simulink library "LDM_Controller"  (R2018b)
settings: Solver=VariableStepAuto  StartTime=0.0  StopTime=10.0  RelTol=1e-3
values from neighbouring files (symbols this model uses):
  K10_LDM_aOLCtrlerTableX : value not decoded    [LDM_DataDict.sldd]
  K10_LDM_torqOLCtrlerTableY : value not decoded    [LDM_DataDict.sldd]
  K_LDM_torqDecelClsCtrlerLowLim = -1000.0    [LDM_DataDict.sldd]
  K_LDM_torqDecelClsCtrlerUpLim = 1000.0    [LDM_DataDict.sldd]
  K_LDM_torqDecelCtrlerLowLim = 0.0    [LDM_DataDict.sldd]
  K_LDM_torqDecelCtrlerUpLim = 20000.0    [LDM_DataDict.sldd]
  K_LDM_torqOLCtrlerDecRate = 2.0    [LDM_DataDict.sldd]
  K_LDM_torqOLCtrlerIncRate = 2.0    [LDM_DataDict.sldd]
  K_LDM_torqOLCtrlerLowLim = 0.0    [LDM_DataDict.sldd]
  K_LDM_torqOLCtrlerResetLim = 10.0    [LDM_DataDict.sldd]
  K_LDM_torqOLCtrlerUpLim = 20000.0    [LDM_DataDict.sldd]
  LDM_VLD_EN_T : value not decoded    [LDM_DataDict.sldd]
  LDMCtrlMode_en_t : value not decoded    [LDM_DataDict.sldd]
undefined symbols (not defined in the file or in its folder): DiscIntNeverNeededParam
libraries: simulink x12
(part 1 of 2)
settings Model: Creator=wxmjy  LastModifiedBy=wxmjy

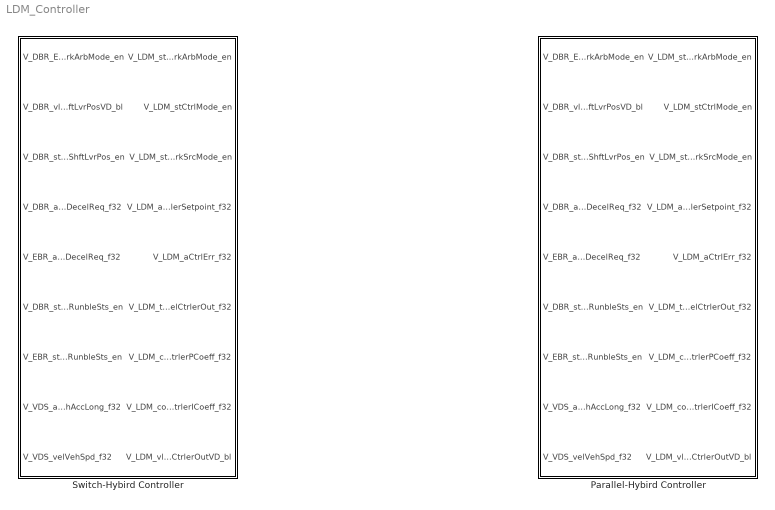
== system LDM_Controller ==
  Parallel-Hybird Controller : Subsystem
  Switch-Hybird Controller : Subsystem

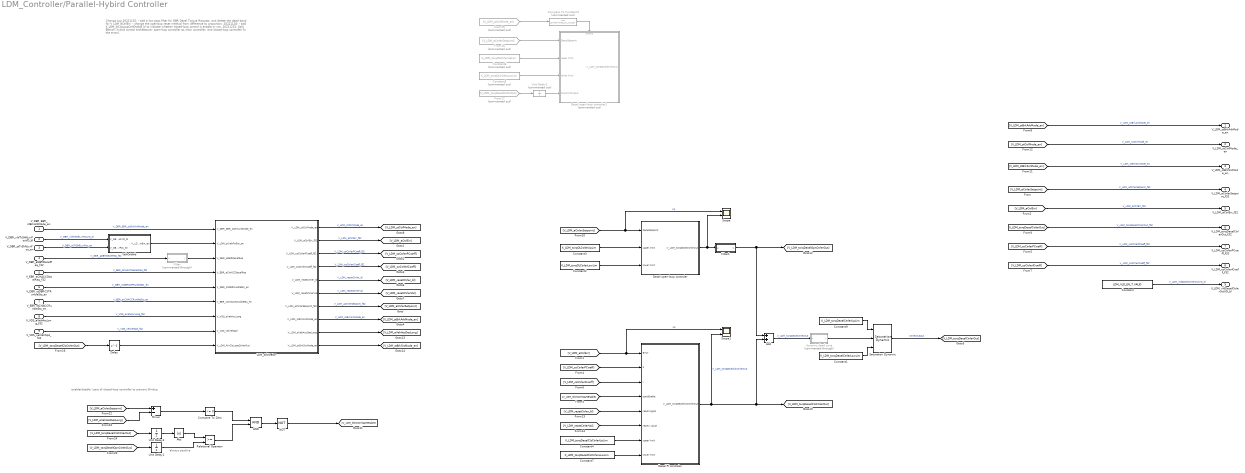
== system LDM_Controller/Parallel-Hybird Controller ==
  note: Change Log
      | 20221125:
      | - add a low-pass filter for DBR Decel Torque Request, and delete the dead band for V_LDM_aCtrlErr;
      | - change the openloop reset method from difference to proportion;
      | 20221128:
      | - add K_LDM_blClsLoopCtrlEnable_bl to indicate whether closed-loop control is enable or not.
      | 20221223:
      | Split Branch: hybrid control architecture: open-loop controller as main controller, and closed-loop controller fix the errors.
  note: always positive
  note: enable/disable I part of closed-loop controller to prevent Windup
  V_DBR_EBR_stBrkArbMode_en : Inport  OutDataTypeStr=Enum: BrkArbMode_en_t
  V_DBR_vldTrShftLvrPosVD_bl : Inport  Port=2
  V_DBR_stTrShftLvrPos_en : Inport  Port=3  OutDataTypeStr=Enum: TrShftLvrPos_en_t
  V_DBR_aDBRDecelReq_f32 : Inport  Port=4
  V_EBR_aCHACCDecelReq_f32 : Inport  Port=5
  V_DBR_stDBRCSTRunbleSts_en : Inport  Port=6  OutDataTypeStr=Enum: DBRCSTRunbleSts_en_t
  V_EBR_stCHACCRunbleSts_en : Inport  Port=7  OutDataTypeStr=Enum: CHACCRunbleSts_en_t
  V_VDS_aVehAccLong_f32 : Inport  Port=8
  V_VDS_velVehSpd_f32 : Inport  Port=9
  AND : Logic  AllPortsSameDT=off  OutDataTypeStr=boolean
  Abs : Abs
  Add : Sum
  Compare To Constant1 : simulink/Logic and Bit Operations/Compare To Constant  Commented=on  relop===  const=LDMCtrlMode_en_t.OLCtrl  OutDataTypeStr=boolean
  Compare To Zero : simulink/Logic and Bit Operations/Compare To Zero  relop=<=  OutDataTypeStr=boolean
  Constant : Constant  Value=LDM_VLD_EN_T.VALID
  Constant1 : Constant  Value=K_LDM_torqDecelCtrlerLowLim  OutDataTypeStr=single
  Constant2 : Constant  Value=K_LDM_torqOLCtrlerLowLim  OutDataTypeStr=single
  Constant3 : Constant  Value=K_LDM_torqOLCtrlerUpLim  OutDataTypeStr=single
  Constant4 : Constant  Value=K_LDM_torqDecelClsCtrlerUpLim  OutDataTypeStr=single
  Constant5 : Constant  Commented=on  Value=K_LDM_torqOLCtrlerLowLim  OutDataTypeStr=single
  Constant6 : Constant  Commented=on  Value=K_LDM_torqOLCtrlerUpLim  OutDataTypeStr=single
  Constant7 : Constant  Value=K_LDM_torqDecelClsCtrlerLowLim  OutDataTypeStr=single
  Constant9 : Constant  Value=K_LDM_torqDecelCtrlerUpLim  OutDataTypeStr=single
  Decel PI controler : Subsystem
  Decel open-loop controler : Subsystem
  Decel open-loop controler1 : Subsystem  Commented=on
  Delay : Delay  DelayLength=1
  Filter : Subsystem  Commented=through
  Filter1 : Subsystem
  From17 : From  Commented=on  GotoTag=V_LDM_torqDecelCtrlerOut
  From18 : From  Commented=on  GotoTag=V_LDM_aCtrlerSetpoint
  From19 : From  Commented=on  GotoTag=V_LDM_stCtrlMode_en
  LDM_Arbitrator : Stateflow chart  TreatAsAtomicUnit=on
  Minus : Sum  Inputs=+-
  NOT : Logic  Operator=NOT  AllPortsSameDT=off  OutDataTypeStr=boolean
  Relational Operator : RelationalOperator  OutDataTypeStr=boolean  RndMeth=Simplest
  Saturation Dynamic : simulink/Discontinuities/Saturation Dynamic  OutMin=[]  OutMax=[]  OutDataTypeStr=single  OutputDataTypeScalingMode=single  OutDataType=fixdt(1, 16)  OutScaling=2^-10  DoSatur=off
  Scope : Scope  NumInputPorts=2
  Scope1 : Scope  NumInputPorts=2
  Unit Delay1 : UnitDelay  SampleTime=-1
  Unit Delay2 : UnitDelay  Commented=on  SampleTime=-1
  Unit Delay3 : UnitDelay  SampleTime=-1
  VehOritArb : Stateflow chart  TreatAsAtomicUnit=on
  dynamic dead zone : Subsystem  Commented=through
  V_LDM_stBrkArbMode_en : Outport
  V_LDM_stCtrlMode_en : Outport  Port=2
  V_LDM_stBrkSrcMode_en : Outport  Port=3
  V_LDM_aCtrlerSetpoint_f32 : Outport  Port=4
  V_LDM_aCtrlErr_f32 : Outport  Port=5
  V_LDM_torqDecelCtrlerOut_f32 : Outport  Port=6
  V_LDM_coCtrlerPCoeff_f32 : Outport  Port=7
  V_LDM_coCtrlerICoeff_f32 : Outport  Port=8
  V_LDM_vldDecelCtrlerOutVD_bl : Outport  Port=9
  wires:
  [V_LDM_stBrkSrcMode_en] -> V_LDM_stBrkSrcMode_en/1  "V_LDM_stBrkSrcMode_en"
  LDM_Arbitrator/10(V_LDM_stBrkSrcMode_en) -> [V_LDM_stBrkSrcMode_en]
  LDM_Arbitrator/9(V_LDM_aVehAccDecLong) -> [V_LDM_aVehAccDecLong]
  Relational Operator/1 -> AND/2
  Compare To Zero/1 -> AND/1
  Minus/1 -> Compare To Zero/1
  [V_LDM_aVehAccDecLong] -> Minus/2
  [V_LDM_aCtrlerSetpoint] -> Minus/1
  NOT/1 -> [V_LDM_blClsCtrlIpartEnable]
  Abs/1 -> Relational Operator/1
  Unit Delay1/1 -> Relational Operator/2
  Unit Delay3/1 -> Abs/1
  [V_LDM_torqDecelClsCtrlerOut] -> Unit Delay3/1
  [V_LDM_torqDecelOpnCtrlerOut] -> Unit Delay1/1
  [V_LDM_blClsCtrlIpartEnable] -> Decel PI controler/4(IpartEnable)
  AND/1 -> NOT/1
  Filter1/1(y) -> Add/1, [V_LDM_torqDecelOpnCtrlerOut]
  Constant/1 -> V_LDM_vldDecelCtrlerOutVD_bl/1  "V_LDM_vldDecelCtrlerOutVD_bl"
  [V_LDM_coCtrlerPCoeff] -> Decel PI controler/2(P)
  Saturation Dynamic/1 -> [V_LDM_torqDecelCtrlerOut]  "CtrlerOutput"
  Constant1/1 -> Saturation Dynamic/3
  Constant9/1 -> Saturation Dynamic/1
  Decel open-loop controler/1(V_LDM_torqDecelCtrlerOut) -> Filter1/1(u), Scope/2
  Decel PI controler/1(V_LDM_torqDecelClsCtrlerOut) -> [V_LDM_torqDecelClsCtrlerOut], Add/2, Scope1/2  "V_LDM_torqDecelClsCtrlerOut"
  [V_LDM_aCtrlErr] -> Decel PI controler/1(Error), Scope1/1  "sp"
  [V_LDM_stBrkArbMode_en] -> V_LDM_stBrkArbMode_en/1  "V_LDM_stBrkArbMode_en"
  LDM_Arbitrator/6(V_LDM_resetCtrlerVal) -> [V_LDM_resetCtrlerVal]  "V_LDM_resetCtrlerVal"
  [V_LDM_coCtrlerICoeff] -> V_LDM_coCtrlerICoeff_f32/1  "V_LDM_coCtrlerICoeff_f32"
  Filter/1(y) -> LDM_Arbitrator/3(V_DBR_aDBRDecelReq)
  [V_LDM_stCtrlMode_en] -> V_LDM_stCtrlMode_en/1  "V_LDM_stCtrlMode_en"
  dynamic dead zone/1(y) -> Saturation Dynamic/2
  [V_LDM_aCtrlerSetpoint] -> Decel open-loop controler/1(DecelSetpoint), Scope/1  "sp"
  [V_LDM_aCtrlerSetpoint] -> V_LDM_aCtrlerSetpoint_f32/1  "V_LDM_aCtrlerSetpoint_f32"
  Constant7/1 -> Decel PI controler/8(lower limit)
  V_DBR_stDBRCSTRunbleSts_en/1 -> LDM_Arbitrator/5(V_DBR_stDBRRunbleSts_en)  "V_DBR_stDBRCSTRunbleSts_en"
  LDM_Arbitrator/2(V_LDM_aCtrlErr_f32) -> [V_LDM_aCtrlErr]  "V_LDM_aCtrlErr_f32"
  LDM_Arbitrator/8(V_LDM_stBrkArbMode_en) -> [V_LDM_stBrkArbMode_en]  "V_LDM_stBrkArbMode_en"
  V_VDS_aVehAccLong_f32/1 -> LDM_Arbitrator/7(V_VDS_aVehAccLong)  "V_VDS_aVehAccLong_f32"
  V_DBR_EBR_stBrkArbMode_en/1 -> LDM_Arbitrator/1(V_DBR_EBR_stBrkArbMode_en)  "V_DBR_EBR_stBrkArbMode_en"
  [V_LDM_torqDecelClsCtrlerOut] -> Delay/1
  [V_LDM_resetCtrlerVal] -> Decel PI controler/6(reset I value)
  V_VDS_velVehSpd_f32/1 -> LDM_Arbitrator/8(V_VDS_velVehSpd)  "V_VDS_velVehSpd_f32"
  Add/1 -> dynamic dead zone/1(u)  "V_LDM_torqDecelCtrlerOut"
  LDM_Arbitrator/1(V_LDM_stCtrlMode_en) -> [V_LDM_stCtrlMode_en]  "V_LDM_stCtrlMode_en"
  V_DBR_stTrShftLvrPos_en/1 -> VehOritArb/2(V_DBR_stTrShftLvrPos_en)  "V_DBR_stTrShftLvrPos_en"
  V_EBR_stCHACCRunbleSts_en/1 -> LDM_Arbitrator/6(V_EBR_stCHACCRunbleSts_en)  "V_EBR_stCHACCRunbleSts_en"
  VehOritArb/1(V_LDM_stVehFwBw_en) -> LDM_Arbitrator/2(V_LDM_stVehFwBw_en)
  Constant4/1 -> Decel PI controler/7(upper limit)
  V_DBR_vldTrShftLvrPosVD_bl/1 -> VehOritArb/1(V_DBR_vldTrShftLvrPosVD_bl)  "V_DBR_vldTrShftLvrPosVD_bl"
  Delay/1 -> LDM_Arbitrator/9(V_LDM_PrvClsLoopCtrlerOut)
  V_DBR_aDBRDecelReq_f32/1 -> Filter/1(u)  "V_DBR_aDBRDecelReq_f32"
  [V_LDM_resetCtrler_bl] -> Decel PI controler/5(reset signal)
  LDM_Arbitrator/3(V_LDM_coCtrlerPCoeff_f32) -> [V_LDM_coCtrlerPCoeff]  "V_LDM_coCtrlerPCoeff_f32"
  Constant2/1 -> Decel open-loop controler/3(lower limit)
  LDM_Arbitrator/4(V_LDM_coCtrlerICoeff_f32) -> [V_LDM_coCtrlerICoeff]  "V_LDM_coCtrlerICoeff_f32"
  [V_LDM_coCtrlerPCoeff] -> V_LDM_coCtrlerPCoeff_f32/1  "V_LDM_coCtrlerPCoeff_f32"
  [V_LDM_aCtrlErr] -> V_LDM_aCtrlErr_f32/1  "V_LDM_aCtrlErr_f32"
  Constant3/1 -> Decel open-loop controler/2(upper limit)
  LDM_Arbitrator/5(V_LDM_resetCtrler_bl) -> [V_LDM_resetCtrler_bl]  "V_LDM_resetCtrler_bl"
  [V_LDM_torqDecelCtrlerOut] -> V_LDM_torqDecelCtrlerOut_f32/1  "V_LDM_torqDecelCtrlerOut_f32"
  V_EBR_aCHACCDecelReq_f32/1 -> LDM_Arbitrator/4(V_EBR_aCHACCDecelReq)  "V_EBR_aCHACCDecelReq_f32"
  LDM_Arbitrator/7(V_LDM_aCtrlerSetpoint_f32) -> [V_LDM_aCtrlerSetpoint]  "V_LDM_aCtrlerSetpoint_f32"
  [V_LDM_coCtrlerICoeff] -> Decel PI controler/3(I)
  Constant6/1 -> Decel open-loop controler1/2(upper limit)
  Constant5/1 -> Decel open-loop controler1/3(lower limit)
  Unit Delay2/1 -> Decel open-loop controler1/4(PrevCtrlOutput)
  From19/1 -> Compare To Constant1/1
  From17/1 -> Unit Delay2/1
  Compare To Constant1/1 -> Decel open-loop controler1/Enable
  From18/1 -> Decel open-loop controler1/1(DecelSetpoint)

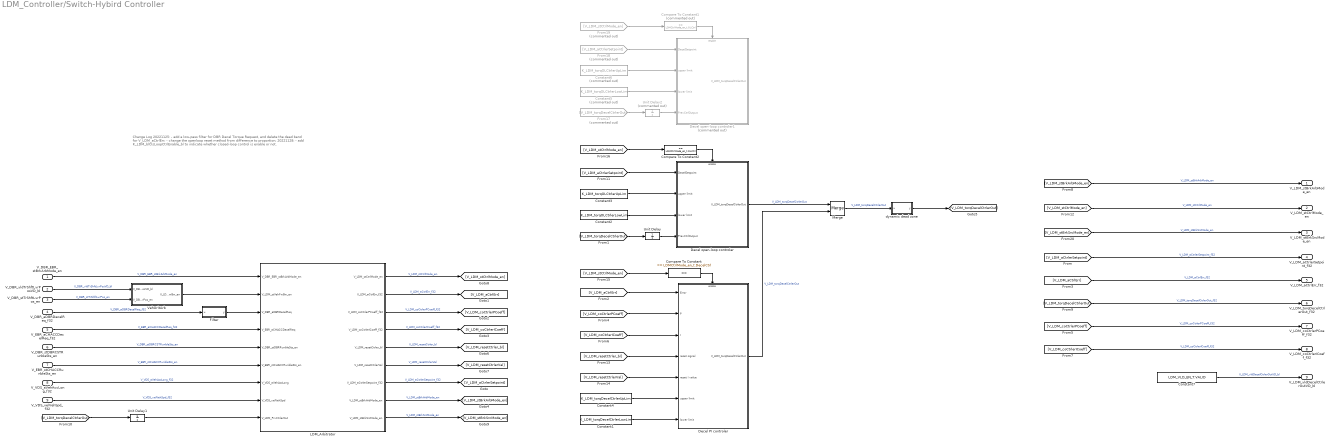
== system LDM_Controller/Switch-Hybird Controller ==
  note: Change Log
      | 20221125:
      | - add a low-pass filter for DBR Decel Torque Request, and delete the dead band for V_LDM_aCtrlErr;
      | - change the openloop reset method from difference to proportion;
      | 20221128:
      | - add K_LDM_blClsLoopCtrlEnable_bl to indicate whether closed-loop control is enable or not.
  V_DBR_EBR_stBrkArbMode_en : Inport  OutDataTypeStr=Enum: BrkArbMode_en_t
  V_DBR_vldTrShftLvrPosVD_bl : Inport  Port=2
  V_DBR_stTrShftLvrPos_en : Inport  Port=3  OutDataTypeStr=Enum: TrShftLvrPos_en_t
  V_DBR_aDBRDecelReq_f32 : Inport  Port=4
  V_EBR_aCHACCDecelReq_f32 : Inport  Port=5
  V_DBR_stDBRCSTRunbleSts_en : Inport  Port=6  OutDataTypeStr=Enum: DBRCSTRunbleSts_en_t
  V_EBR_stCHACCRunbleSts_en : Inport  Port=7  OutDataTypeStr=Enum: CHACCRunbleSts_en_t
  V_VDS_aVehAccLong_f32 : Inport  Port=8
  V_VDS_velVehSpd_f32 : Inport  Port=9
  Compare To Constant : simulink/Logic and Bit Operations/Compare To Constant  relop===  const=LDMCtrlMode_en_t.DecelCtrl  OutDataTypeStr=boolean
  Compare To Constant1 : simulink/Logic and Bit Operations/Compare To Constant  Commented=on  relop===  const=LDMCtrlMode_en_t.OLCtrl  OutDataTypeStr=boolean
  Compare To Constant2 : simulink/Logic and Bit Operations/Compare To Constant  relop===  const=LDMCtrlMode_en_t.OLCtrl  OutDataTypeStr=boolean
  Constant1 : Constant  Value=K_LDM_torqDecelCtrlerLowLim  OutDataTypeStr=single
  Constant2 : Constant  Value=K_LDM_torqOLCtrlerLowLim  OutDataTypeStr=single
  Constant3 : Constant  Value=K_LDM_torqOLCtrlerUpLim  OutDataTypeStr=single
  Constant4 : Constant  Value=K_LDM_torqDecelCtrlerUpLim  OutDataTypeStr=single
  Constant5 : Constant  Commented=on  Value=K_LDM_torqOLCtrlerLowLim  OutDataTypeStr=single
  Constant6 : Constant  Commented=on  Value=K_LDM_torqOLCtrlerUpLim  OutDataTypeStr=single
  Constant7 : Constant  Value=LDM_VLD_EN_T.VALID
  Decel PI controler : Subsystem
  Decel open-loop controler : Subsystem
  Decel open-loop controler1 : Subsystem  Commented=on
  Filter : Subsystem
  From17 : From  Commented=on  GotoTag=V_LDM_torqDecelCtrlerOut
  From18 : From  Commented=on  GotoTag=V_LDM_aCtrlerSetpoint
  From19 : From  Commented=on  GotoTag=V_LDM_stCtrlMode_en
  LDM_Arbitrator : Stateflow chart  TreatAsAtomicUnit=on
  Merge : Merge
  Unit Delay : UnitDelay  SampleTime=-1
  Unit Delay1 : UnitDelay  SampleTime=-1
  Unit Delay2 : UnitDelay  Commented=on  SampleTime=-1
  VehOritArb : Stateflow chart  TreatAsAtomicUnit=on
  dynamic dead zone : Subsystem
  V_LDM_stBrkArbMode_en : Outport
  V_LDM_stCtrlMode_en : Outport  Port=2
  V_LDM_stBrkSrcMode_en : Outport  Port=3
  V_LDM_aCtrlerSetpoint_f32 : Outport  Port=4
  V_LDM_aCtrlErr_f32 : Outport  Port=5
  V_LDM_torqDecelCtrlerOut_f32 : Outport  Port=6
  V_LDM_coCtrlerPCoeff_f32 : Outport  Port=7
  V_LDM_coCtrlerICoeff_f32 : Outport  Port=8
  V_LDM_vldDecelCtrlerOutVD_bl : Outport  Port=9
  wires:
  LDM_Arbitrator/9(V_LDM_stBrkSrcMode_en) -> [V_LDM_stBrkSrcMode_en]  "V_LDM_stBrkSrcMode_en"
  [V_LDM_stBrkSrcMode_en] -> V_LDM_stBrkSrcMode_en/1  "V_LDM_stBrkSrcMode_en"
  Constant7/1 -> V_LDM_vldDecelCtrlerOutVD_bl/1  "V_LDM_vldDecelCtrlerOutVD_bl"
  From18/1 -> Decel open-loop controler1/1(DecelSetpoint)
  Compare To Constant1/1 -> Decel open-loop controler1/Enable
  From17/1 -> Unit Delay2/1
  From19/1 -> Compare To Constant1/1
  Unit Delay2/1 -> Decel open-loop controler1/4(PrevCtrlOutput)
  Constant5/1 -> Decel open-loop controler1/3(lower limit)
  Constant6/1 -> Decel open-loop controler1/2(upper limit)
  [V_LDM_coCtrlerICoeff] -> Decel PI controler/3(I)
  LDM_Arbitrator/7(V_LDM_aCtrlerSetpoint_f32) -> [V_LDM_aCtrlerSetpoint]  "V_LDM_aCtrlerSetpoint_f32"
  V_EBR_aCHACCDecelReq_f32/1 -> LDM_Arbitrator/4(V_EBR_aCHACCDecelReq)  "V_EBR_aCHACCDecelReq_f32"
  [V_LDM_torqDecelCtrlerOut] -> V_LDM_torqDecelCtrlerOut_f32/1  "V_LDM_torqDecelCtrlerOut_f32"
  LDM_Arbitrator/5(V_LDM_resetCtrler_bl) -> [V_LDM_resetCtrler_bl]  "V_LDM_resetCtrler_bl"
  [V_LDM_stCtrlMode_en] -> Compare To Constant/1
  Constant3/1 -> Decel open-loop controler/2(upper limit)
  [V_LDM_aCtrlErr] -> Decel PI controler/1(Error)
  [V_LDM_aCtrlErr] -> V_LDM_aCtrlErr_f32/1  "V_LDM_aCtrlErr_f32"
  [V_LDM_coCtrlerPCoeff] -> V_LDM_coCtrlerPCoeff_f32/1  "V_LDM_coCtrlerPCoeff_f32"
  [V_LDM_coCtrlerICoeff] -> V_LDM_coCtrlerICoeff_f32/1  "V_LDM_coCtrlerICoeff_f32"
  LDM_Arbitrator/4(V_LDM_coCtrlerICoeff_f32) -> [V_LDM_coCtrlerICoeff]  "V_LDM_coCtrlerICoeff_f32"
  [V_LDM_coCtrlerPCoeff] -> Decel PI controler/2(P)
  Constant2/1 -> Decel open-loop controler/3(lower limit)
  LDM_Arbitrator/3(V_LDM_coCtrlerPCoeff_f32) -> [V_LDM_coCtrlerPCoeff]  "V_LDM_coCtrlerPCoeff_f32"
  [V_LDM_resetCtrler_bl] -> Decel PI controler/4(reset signal)
  V_DBR_aDBRDecelReq_f32/1 -> Filter/1(u)  "V_DBR_aDBRDecelReq_f32"
  Merge/1 -> dynamic dead zone/1(u)  "V_LDM_torqDecelCtrlerOut"
  Unit Delay1/1 -> LDM_Arbitrator/9(V_LDM_PrvCtrlerOut)
  V_DBR_vldTrShftLvrPosVD_bl/1 -> VehOritArb/1(V_DBR_vldTrShftLvrPosVD_bl)  "V_DBR_vldTrShftLvrPosVD_bl"
  Constant4/1 -> Decel PI controler/6(upper limit)
  VehOritArb/1(V_LDM_stVehFwBw_en) -> LDM_Arbitrator/2(V_LDM_stVehFwBw_en)
  V_EBR_stCHACCRunbleSts_en/1 -> LDM_Arbitrator/6(V_EBR_stCHACCRunbleSts_en)  "V_EBR_stCHACCRunbleSts_en"
  V_DBR_stTrShftLvrPos_en/1 -> VehOritArb/2(V_DBR_stTrShftLvrPos_en)  "V_DBR_stTrShftLvrPos_en"
  LDM_Arbitrator/1(V_LDM_stCtrlMode_en) -> [V_LDM_stCtrlMode_en]  "V_LDM_stCtrlMode_en"
  Unit Delay/1 -> Decel open-loop controler/4(PrevCtrlOutput)
  Decel PI controler/1(V_LDM_torqDecelCtrlerOut) -> Merge/2  "V_LDM_torqDecelCtrlerOut"
  V_VDS_velVehSpd_f32/1 -> LDM_Arbitrator/8(V_VDS_velVehSpd)  "V_VDS_velVehSpd_f32"
  [V_LDM_resetCtrlerVal] -> Decel PI controler/5(reset I value)
  [V_LDM_torqDecelCtrlerOut] -> Unit Delay1/1
  Decel open-loop controler/1(V_LDM_torqDecelCtrlerOut) -> Merge/1  "V_LDM_torqDecelCtrlerOut"
  V_DBR_EBR_stBrkArbMode_en/1 -> LDM_Arbitrator/1(V_DBR_EBR_stBrkArbMode_en)  "V_DBR_EBR_stBrkArbMode_en"
  [V_LDM_stCtrlMode_en] -> Compare To Constant2/1
  [V_LDM_torqDecelCtrlerOut] -> Unit Delay/1
  V_VDS_aVehAccLong_f32/1 -> LDM_Arbitrator/7(V_VDS_aVehAccLong)  "V_VDS_aVehAccLong_f32"
  LDM_Arbitrator/8(V_LDM_stBrkArbMode_en) -> [V_LDM_stBrkArbMode_en]  "V_LDM_stBrkArbMode_en"
  LDM_Arbitrator/2(V_LDM_aCtrlErr_f32) -> [V_LDM_aCtrlErr]  "V_LDM_aCtrlErr_f32"
  V_DBR_stDBRCSTRunbleSts_en/1 -> LDM_Arbitrator/5(V_DBR_stDBRRunbleSts_en)  "V_DBR_stDBRCSTRunbleSts_en"
  Compare To Constant/1 -> Decel PI controler/Enable
  Constant1/1 -> Decel PI controler/7(lower limit)
  Compare To Constant2/1 -> Decel open-loop controler/Enable
  [V_LDM_aCtrlerSetpoint] -> V_LDM_aCtrlerSetpoint_f32/1  "V_LDM_aCtrlerSetpoint_f32"
  [V_LDM_aCtrlerSetpoint] -> Decel open-loop controler/1(DecelSetpoint)
  dynamic dead zone/1(y) -> [V_LDM_torqDecelCtrlerOut]
  [V_LDM_stCtrlMode_en] -> V_LDM_stCtrlMode_en/1  "V_LDM_stCtrlMode_en"
  Filter/1(y) -> LDM_Arbitrator/3(V_DBR_aDBRDecelReq)
  LDM_Arbitrator/6(V_LDM_resetCtrlerVal) -> [V_LDM_resetCtrlerVal]  "V_LDM_resetCtrlerVal"
  [V_LDM_stBrkArbMode_en] -> V_LDM_stBrkArbMode_en/1  "V_LDM_stBrkArbMode_en"

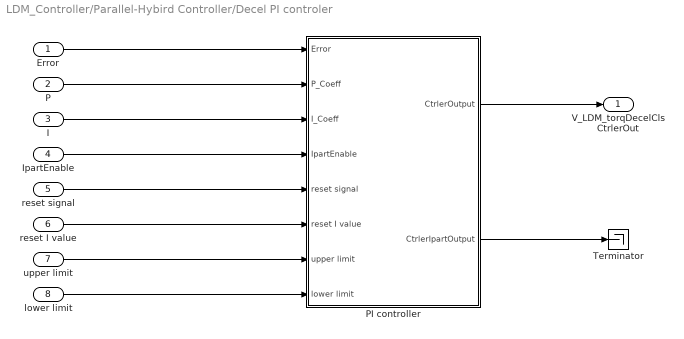
== system LDM_Controller/Parallel-Hybird Controller/Decel PI controler ==
  Error : Inport
  P : Inport  Port=2
  I : Inport  Port=3
  IpartEnable : Inport  Port=4
  reset signal : Inport  Port=5
  reset I value : Inport  Port=6
  upper limit : Inport  Port=7
  lower limit : Inport  Port=8
  PI controller : Subsystem
  Terminator : Terminator
  V_LDM_torqDecelClsCtrlerOut : Outport
  wires:
  IpartEnable/1 -> PI controller/4(IpartEnable)
  PI controller/2(CtrlerIpartOutput) -> Terminator/1
  Error/1 -> PI controller/1(Error)
  P/1 -> PI controller/2(P_Coeff)
  I/1 -> PI controller/3(I_Coeff)
  reset signal/1 -> PI controller/5(reset signal)
  reset I value/1 -> PI controller/6(reset I value)
  PI controller/1(CtrlerOutput) -> V_LDM_torqDecelClsCtrlerOut/1
  lower limit/1 -> PI controller/8(lower limit)
  upper limit/1 -> PI controller/7(upper limit)

== system LDM_Controller/Parallel-Hybird Controller/Decel open-loop controler ==
  DecelSetpoint : Inport
  upper limit : Inport  Port=2
  lower limit : Inport  Port=3
  2-D Lookup Table1 : Lookup_n-D  NumberOfTableDimensions=1  BreakpointsForDimension1=K10_LDM_aOLCtrlerTableX  BreakpointsForDimension2=[0.1,0.2,0.3]  Table=K10_LDM_torqOLCtrlerTableY  InternalRulePriority=Speed  RndMeth=Simplest  InputSameDT=on
  Saturation Dynamic : simulink/Discontinuities/Saturation Dynamic  OutMin=[]  OutMax=[]  OutDataTypeStr=single  OutputDataTypeScalingMode=single  OutDataType=fixdt(1, 16)  OutScaling=2^-10  DoSatur=off
  Signal Conversion : SignalConversion  OverrideOpt=off
  V_LDM_torqDecelCtrlerOut : Outport
  wires:
  DecelSetpoint/1 -> 2-D Lookup Table1/1
  upper limit/1 -> Saturation Dynamic/1
  lower limit/1 -> Saturation Dynamic/3
  Saturation Dynamic/1 -> Signal Conversion/1
  Signal Conversion/1 -> V_LDM_torqDecelCtrlerOut/1
  2-D Lookup Table1/1 -> Saturation Dynamic/2

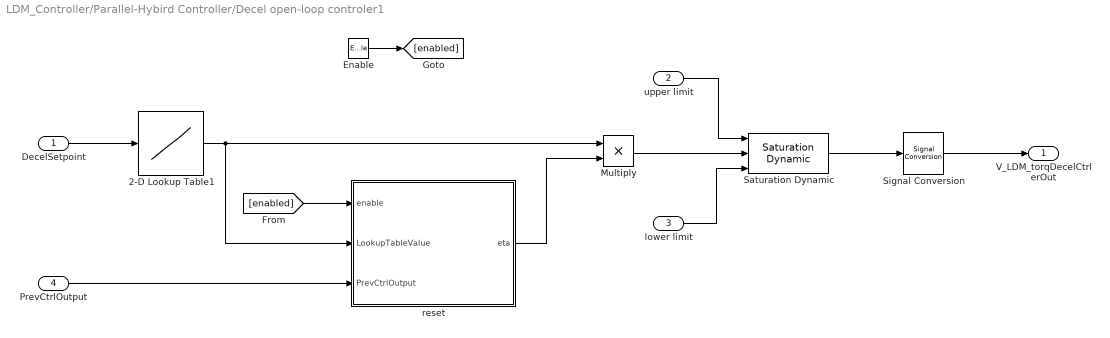
== system LDM_Controller/Parallel-Hybird Controller/Decel open-loop controler1 ==
  DecelSetpoint : Inport
  upper limit : Inport  Port=2
  lower limit : Inport  Port=3
  PrevCtrlOutput : Inport  Port=4
  Enable : EnablePort  ShowOutputPort=on
  2-D Lookup Table1 : Lookup_n-D  NumberOfTableDimensions=1  BreakpointsForDimension1=K10_LDM_aOLCtrlerTableX  BreakpointsForDimension2=[0.1,0.2,0.3]  Table=K10_LDM_torqOLCtrlerTableY  InternalRulePriority=Speed  RndMeth=Simplest  InputSameDT=on
  Multiply : Product
  Saturation Dynamic : simulink/Discontinuities/Saturation Dynamic  OutMin=[]  OutMax=[]  OutDataTypeStr=single  OutputDataTypeScalingMode=single  OutDataType=fixdt(1, 16)  OutScaling=2^-10  DoSatur=off
  Signal Conversion : SignalConversion  OverrideOpt=off
  reset : Stateflow chart  TreatAsAtomicUnit=on
  V_LDM_torqDecelCtrlerOut : Outport
  wires:
  [enabled] -> reset/1(enable)
  Multiply/1 -> Saturation Dynamic/2
  reset/1(eta) -> Multiply/2
  PrevCtrlOutput/1 -> reset/3(PrevCtrlOutput)
  Enable/1 -> [enabled]
  DecelSetpoint/1 -> 2-D Lookup Table1/1
  Signal Conversion/1 -> V_LDM_torqDecelCtrlerOut/1
  Saturation Dynamic/1 -> Signal Conversion/1
  lower limit/1 -> Saturation Dynamic/3
  upper limit/1 -> Saturation Dynamic/1
  2-D Lookup Table1/1 -> reset/2(LookupTableValue), Multiply/1

== system LDM_Controller/Parallel-Hybird Controller/Filter ==
  u : Inport
  Add : Sum
  Constant1 : Constant  Value=0.5  OutDataTypeStr=single
  Constant2 : Constant  OutDataTypeStr=single
  Minus : Sum  Inputs=+-
  Multiply : Product
  Multiply1 : Product
  Unit Delay : UnitDelay  SampleTime=-1
  y : Outport
  wires:
  Constant2/1 -> Minus/1
  Minus/1 -> Multiply1/2
  Add/1 -> y/1, Unit Delay/1  "y"
  Unit Delay/1 -> Multiply/2  "y_k-1"
  Multiply1/1 -> Add/1
  Multiply/1 -> Add/2
  Constant1/1 -> Multiply/1, Minus/2
  u/1 -> Multiply1/1

== system LDM_Controller/Parallel-Hybird Controller/Filter1 ==
  u : Inport
  Add : Sum
  Constant1 : Constant  Value=0.7  OutDataTypeStr=single
  Constant2 : Constant  Value=0.3  OutDataTypeStr=single
  Multiply : Product
  Multiply1 : Product
  Unit Delay : UnitDelay  SampleTime=-1
  y : Outport
  wires:
  Constant2/1 -> Multiply1/2
  Add/1 -> y/1, Unit Delay/1  "y"
  Unit Delay/1 -> Multiply/2  "y_k-1"
  Multiply1/1 -> Add/1
  Multiply/1 -> Add/2
  Constant1/1 -> Multiply/1
  u/1 -> Multiply1/1

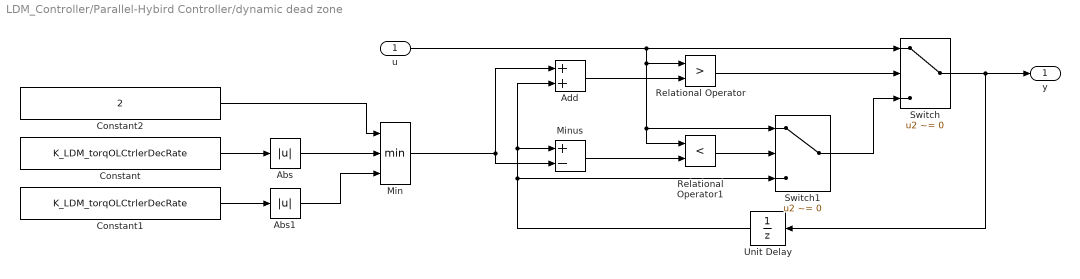
== system LDM_Controller/Parallel-Hybird Controller/dynamic dead zone ==
  u : Inport
  Abs : Abs
  Abs1 : Abs
  Add : Sum
  Constant : Constant  Value=K_LDM_torqOLCtrlerDecRate  OutDataTypeStr=single
  Constant1 : Constant  Value=K_LDM_torqOLCtrlerDecRate  OutDataTypeStr=single
  Constant2 : Constant  Value=2  OutDataTypeStr=single
  Min : MinMax  Inputs=3
  Minus : Sum  Inputs=+-
  Relational Operator : RelationalOperator  Operator=>  OutDataTypeStr=boolean  RndMeth=Simplest
  Relational Operator1 : RelationalOperator  Operator=<  OutDataTypeStr=boolean  RndMeth=Simplest
  Switch : Switch  Criteria=u2 ~= 0
  Switch1 : Switch  Criteria=u2 ~= 0
  Unit Delay : UnitDelay  SampleTime=-1
  y : Outport
  wires:
  Switch/1 -> Unit Delay/1, y/1
  u/1 -> Switch/1, Relational Operator1/1, Switch1/1, Relational Operator/1
  Unit Delay/1 -> Minus/1, Add/2, Switch1/3
  Constant/1 -> Abs/1
  Add/1 -> Relational Operator/2
  Minus/1 -> Relational Operator1/2
  Relational Operator/1 -> Switch/2
  Relational Operator1/1 -> Switch1/2
  Switch1/1 -> Switch/3
  Min/1 -> Add/1, Minus/2
  Constant1/1 -> Abs1/1
  Abs/1 -> Min/2
  Abs1/1 -> Min/3
  Constant2/1 -> Min/1

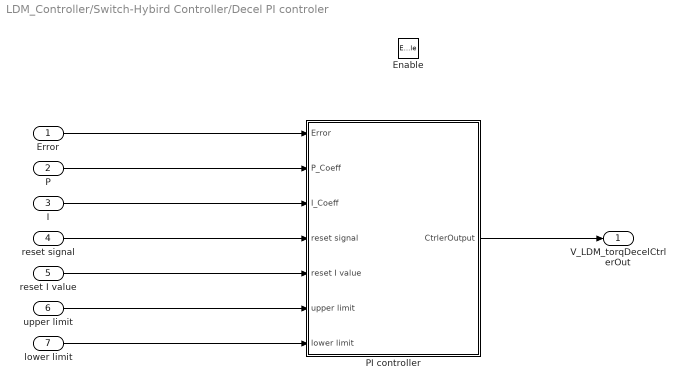
== system LDM_Controller/Switch-Hybird Controller/Decel PI controler ==
  Error : Inport
  P : Inport  Port=2
  I : Inport  Port=3
  reset signal : Inport  Port=4
  reset I value : Inport  Port=5
  upper limit : Inport  Port=6
  lower limit : Inport  Port=7
  Enable : EnablePort
  PI controller : Subsystem
  V_LDM_torqDecelCtrlerOut : Outport
  wires:
  upper limit/1 -> PI controller/6(upper limit)
  lower limit/1 -> PI controller/7(lower limit)
  PI controller/1(CtrlerOutput) -> V_LDM_torqDecelCtrlerOut/1
  reset I value/1 -> PI controller/5(reset I value)
  reset signal/1 -> PI controller/4(reset signal)
  I/1 -> PI controller/3(I_Coeff)
  P/1 -> PI controller/2(P_Coeff)
  Error/1 -> PI controller/1(Error)

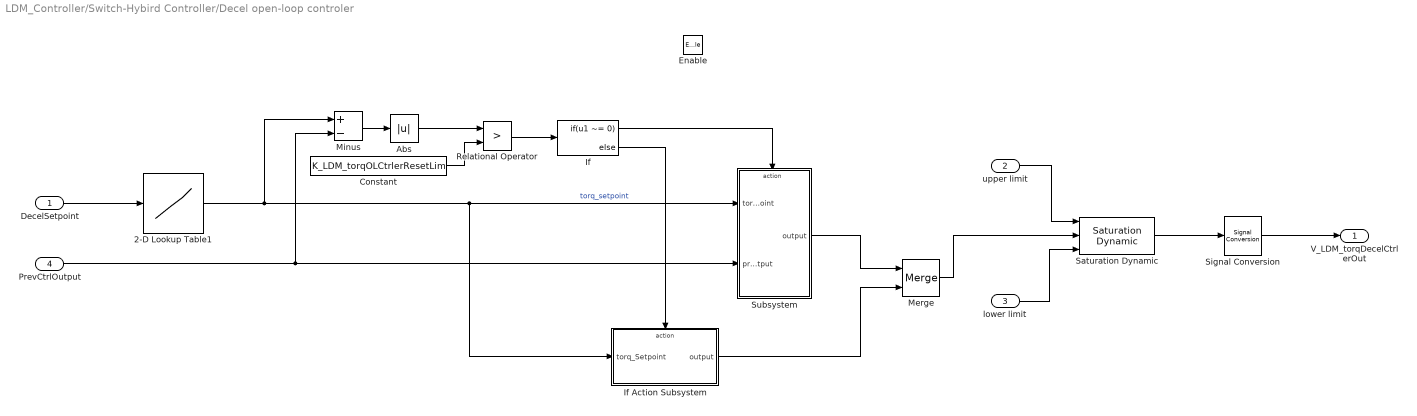
== system LDM_Controller/Switch-Hybird Controller/Decel open-loop controler ==
  DecelSetpoint : Inport
  upper limit : Inport  Port=2
  lower limit : Inport  Port=3
  PrevCtrlOutput : Inport  Port=4
  Enable : EnablePort
  2-D Lookup Table1 : Lookup_n-D  NumberOfTableDimensions=1  BreakpointsForDimension1=K10_LDM_aOLCtrlerTableX  BreakpointsForDimension2=[0.1,0.2,0.3]  Table=K10_LDM_torqOLCtrlerTableY  InternalRulePriority=Speed  RndMeth=Simplest  InputSameDT=on
  Abs : Abs
  Constant : Constant  Value=K_LDM_torqOLCtrlerResetLim  OutDataTypeStr=single
  If : If  IfExpression=u1 ~= 0
  If Action Subsystem : Subsystem  TreatAsAtomicUnit=on
  Merge : Merge
  Minus : Sum  Inputs=+-
  Relational Operator : RelationalOperator  Operator=>  OutDataTypeStr=boolean  RndMeth=Simplest
  Saturation Dynamic : simulink/Discontinuities/Saturation Dynamic  OutMin=[]  OutMax=[]  OutDataTypeStr=single  OutputDataTypeScalingMode=single  OutDataType=fixdt(1, 16)  OutScaling=2^-10  DoSatur=off
  Signal Conversion : SignalConversion  OverrideOpt=off
  Subsystem : Subsystem
  V_LDM_torqDecelCtrlerOut : Outport
  wires:
  If Action Subsystem/1(output) -> Merge/2
  Subsystem/1(output) -> Merge/1
  If/2 -> If Action Subsystem/Action
  Constant/1 -> Relational Operator/2
  Relational Operator/1 -> If/1
  If/1 -> Subsystem/Action
  Merge/1 -> Saturation Dynamic/2
  Abs/1 -> Relational Operator/1
  Minus/1 -> Abs/1
  2-D Lookup Table1/1 -> Subsystem/1(torq_setpoint), If Action Subsystem/1(torq_Setpoint), Minus/1  "torq_setpoint"
  PrevCtrlOutput/1 -> Subsystem/2(prevOutput), Minus/2
  Signal Conversion/1 -> V_LDM_torqDecelCtrlerOut/1
  Saturation Dynamic/1 -> Signal Conversion/1
  lower limit/1 -> Saturation Dynamic/3
  upper limit/1 -> Saturation Dynamic/1
  DecelSetpoint/1 -> 2-D Lookup Table1/1

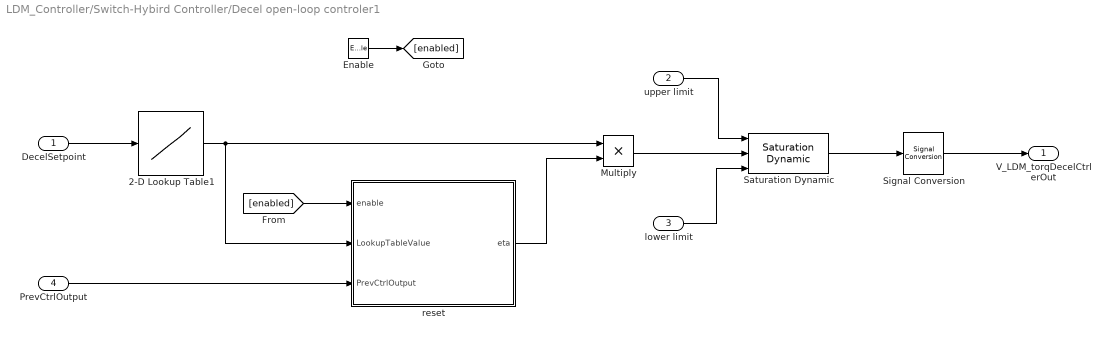
== system LDM_Controller/Switch-Hybird Controller/Decel open-loop controler1 ==
  DecelSetpoint : Inport
  upper limit : Inport  Port=2
  lower limit : Inport  Port=3
  PrevCtrlOutput : Inport  Port=4
  Enable : EnablePort  ShowOutputPort=on
  2-D Lookup Table1 : Lookup_n-D  NumberOfTableDimensions=1  BreakpointsForDimension1=K10_LDM_aOLCtrlerTableX  BreakpointsForDimension2=[0.1,0.2,0.3]  Table=K10_LDM_torqOLCtrlerTableY  InternalRulePriority=Speed  RndMeth=Simplest  InputSameDT=on
  Multiply : Product
  Saturation Dynamic : simulink/Discontinuities/Saturation Dynamic  OutMin=[]  OutMax=[]  OutDataTypeStr=single  OutputDataTypeScalingMode=single  OutDataType=fixdt(1, 16)  OutScaling=2^-10  DoSatur=off
  Signal Conversion : SignalConversion  OverrideOpt=off
  reset : Stateflow chart  TreatAsAtomicUnit=on
  V_LDM_torqDecelCtrlerOut : Outport
  wires:
  2-D Lookup Table1/1 -> Multiply/1, reset/2(LookupTableValue)
  upper limit/1 -> Saturation Dynamic/1
  lower limit/1 -> Saturation Dynamic/3
  Saturation Dynamic/1 -> Signal Conversion/1
  Signal Conversion/1 -> V_LDM_torqDecelCtrlerOut/1
  DecelSetpoint/1 -> 2-D Lookup Table1/1
  Enable/1 -> [enabled]
  PrevCtrlOutput/1 -> reset/3(PrevCtrlOutput)
  reset/1(eta) -> Multiply/2
  Multiply/1 -> Saturation Dynamic/2
  [enabled] -> reset/1(enable)

== system LDM_Controller/Switch-Hybird Controller/Filter ==
  u : Inport
  Add : Sum
  Constant1 : Constant  Value=0.5  OutDataTypeStr=single
  Constant2 : Constant  OutDataTypeStr=single
  Minus : Sum  Inputs=+-
  Multiply : Product
  Multiply1 : Product
  Unit Delay : UnitDelay  SampleTime=-1
  y : Outport
  wires:
  u/1 -> Multiply1/1
  Constant1/1 -> Minus/2, Multiply/1
  Multiply/1 -> Add/2
  Multiply1/1 -> Add/1
  Unit Delay/1 -> Multiply/2  "y_k-1"
  Add/1 -> Unit Delay/1, y/1  "y"
  Minus/1 -> Multiply1/2
  Constant2/1 -> Minus/1

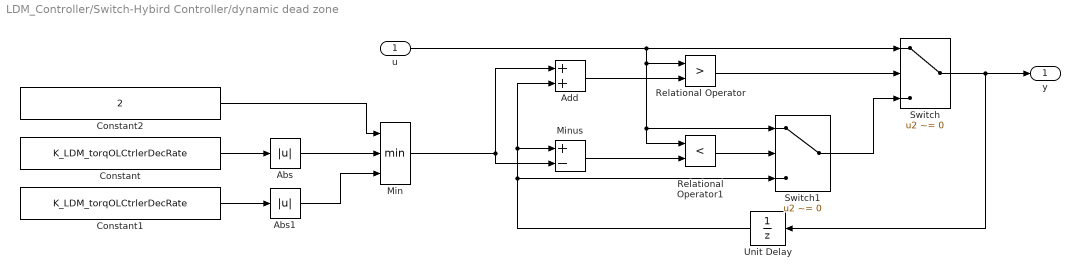
== system LDM_Controller/Switch-Hybird Controller/dynamic dead zone ==
  u : Inport
  Abs : Abs
  Abs1 : Abs
  Add : Sum
  Constant : Constant  Value=K_LDM_torqOLCtrlerDecRate  OutDataTypeStr=single
  Constant1 : Constant  Value=K_LDM_torqOLCtrlerDecRate  OutDataTypeStr=single
  Constant2 : Constant  Value=2  OutDataTypeStr=single
  Min : MinMax  Inputs=3
  Minus : Sum  Inputs=+-
  Relational Operator : RelationalOperator  Operator=>  OutDataTypeStr=boolean  RndMeth=Simplest
  Relational Operator1 : RelationalOperator  Operator=<  OutDataTypeStr=boolean  RndMeth=Simplest
  Switch : Switch  Criteria=u2 ~= 0
  Switch1 : Switch  Criteria=u2 ~= 0
  Unit Delay : UnitDelay  SampleTime=-1
  y : Outport
  wires:
  Constant2/1 -> Min/1
  Abs1/1 -> Min/3
  Abs/1 -> Min/2
  Constant1/1 -> Abs1/1
  Min/1 -> Minus/2, Add/1
  Switch1/1 -> Switch/3
  Relational Operator1/1 -> Switch1/2
  Relational Operator/1 -> Switch/2
  Minus/1 -> Relational Operator1/2
  Add/1 -> Relational Operator/2
  Constant/1 -> Abs/1
  Unit Delay/1 -> Switch1/3, Add/2, Minus/1
  u/1 -> Relational Operator/1, Switch1/1, Relational Operator1/1, Switch/1
  Switch/1 -> y/1, Unit Delay/1

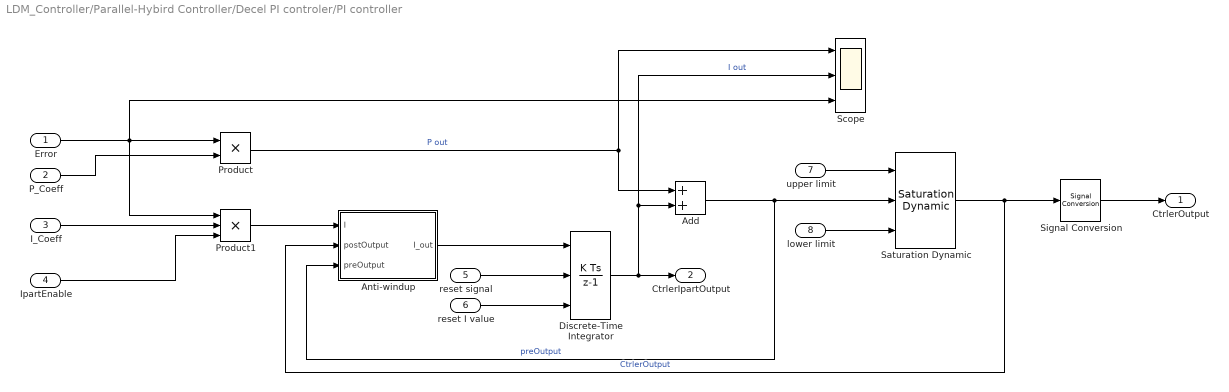
== system LDM_Controller/Parallel-Hybird Controller/Decel PI controler/PI controller ==
  Error : Inport
  P_Coeff : Inport  Port=2
  I_Coeff : Inport  Port=3
  IpartEnable : Inport  Port=4
  reset signal : Inport  Port=5
  reset I value : Inport  Port=6
  upper limit : Inport  Port=7
  lower limit : Inport  Port=8
  Add : Sum
  Anti-windup : Subsystem
  Discrete-Time Integrator : DiscreteIntegrator  ExternalReset=either  InitialConditionSource=external  SampleTime=-1  ICPrevOutput=DiscIntNeverNeededParam  ICPrevScaledInput=DiscIntNeverNeededParam
  Product : Product  OutDataTypeStr=Inherit: Same as first input
  Product1 : Product  Inputs=3  OutDataTypeStr=Inherit: Same as first input
  Saturation Dynamic : simulink/Discontinuities/Saturation Dynamic  OutMin=[]  OutMax=[]  OutDataTypeStr=single  OutputDataTypeScalingMode=single  OutDataType=fixdt(1, 16)  OutScaling=2^-10  DoSatur=off
  Scope : Scope  NumInputPorts=3
  Signal Conversion : SignalConversion  OverrideOpt=off
  CtrlerOutput : Outport
  CtrlerIpartOutput : Outport  Port=2
  wires:
  IpartEnable/1 -> Product1/3
  Add/1 -> Saturation Dynamic/2, Anti-windup/3(preOutput)  "preOutput"
  reset I value/1 -> Discrete-Time Integrator/3
  reset signal/1 -> Discrete-Time Integrator/2
  Product/1 -> Scope/1, Add/1  "P out"
  Product1/1 -> Anti-windup/1(I)
  Discrete-Time Integrator/1 -> CtrlerIpartOutput/1, Scope/2, Add/2  "I out"
  lower limit/1 -> Saturation Dynamic/3
  Error/1 -> Product/1, Product1/1, Scope/3
  Saturation Dynamic/1 -> Signal Conversion/1, Anti-windup/2(postOutput)  "CtrlerOutput"
  P_Coeff/1 -> Product/2
  I_Coeff/1 -> Product1/2
  upper limit/1 -> Saturation Dynamic/1
  Signal Conversion/1 -> CtrlerOutput/1
  Anti-windup/1(I_out) -> Discrete-Time Integrator/1

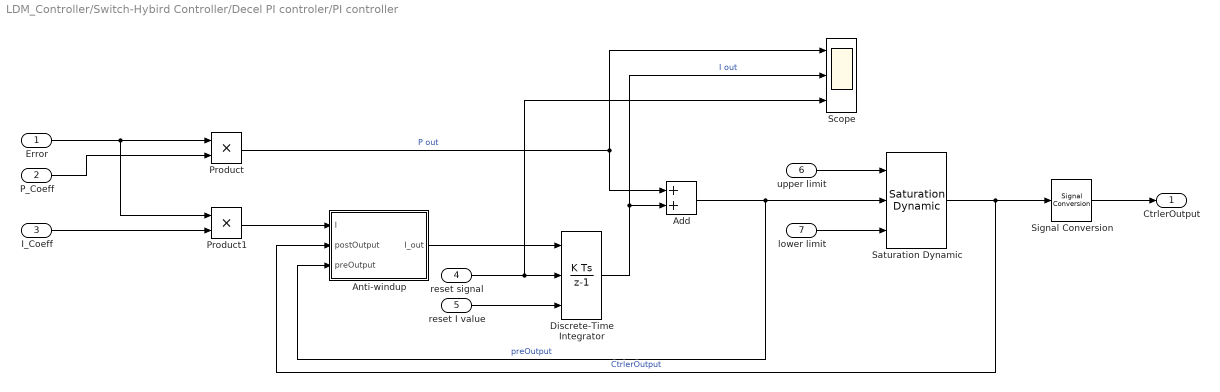
== system LDM_Controller/Switch-Hybird Controller/Decel PI controler/PI controller ==
  Error : Inport
  P_Coeff : Inport  Port=2
  I_Coeff : Inport  Port=3
  reset signal : Inport  Port=4
  reset I value : Inport  Port=5
  upper limit : Inport  Port=6
  lower limit : Inport  Port=7
  Add : Sum
  Anti-windup : Subsystem
  Discrete-Time Integrator : DiscreteIntegrator  ExternalReset=either  InitialConditionSource=external  SampleTime=-1  ICPrevOutput=DiscIntNeverNeededParam  ICPrevScaledInput=DiscIntNeverNeededParam
  Product : Product  OutDataTypeStr=Inherit: Same as first input
  Product1 : Product  OutDataTypeStr=Inherit: Same as first input
  Saturation Dynamic : simulink/Discontinuities/Saturation Dynamic  OutMin=[]  OutMax=[]  OutDataTypeStr=single  OutputDataTypeScalingMode=single  OutDataType=fixdt(1, 16)  OutScaling=2^-10  DoSatur=off
  Scope : Scope  NumInputPorts=3
  Signal Conversion : SignalConversion  OverrideOpt=off
  CtrlerOutput : Outport
  wires:
  Anti-windup/1(I_out) -> Discrete-Time Integrator/1
  Signal Conversion/1 -> CtrlerOutput/1
  upper limit/1 -> Saturation Dynamic/1
  I_Coeff/1 -> Product1/2
  P_Coeff/1 -> Product/2
  Saturation Dynamic/1 -> Anti-windup/2(postOutput), Signal Conversion/1  "CtrlerOutput"
  Error/1 -> Product1/1, Product/1
  lower limit/1 -> Saturation Dynamic/3
  Discrete-Time Integrator/1 -> Add/2, Scope/2  "I out"
  Product1/1 -> Anti-windup/1(I)
  Product/1 -> Add/1, Scope/1  "P out"
  reset signal/1 -> Discrete-Time Integrator/2, Scope/3
  reset I value/1 -> Discrete-Time Integrator/3
  Add/1 -> Anti-windup/3(preOutput), Saturation Dynamic/2  "preOutput"

== system LDM_Controller/Switch-Hybird Controller/Decel open-loop controler/If Action Subsystem ==
  torq_Setpoint : Inport
  Action Port : ActionPort
  output : Outport
  wires:
  torq_Setpoint/1 -> output/1

== system LDM_Controller/Switch-Hybird Controller/Decel open-loop controler/Subsystem ==
  torq_setpoint : Inport
  prevOutput : Inport  Port=2
  Action Port : ActionPort
  Chart : Stateflow chart  TreatAsAtomicUnit=on
  output : Outport
  wires:
  prevOutput/1 -> Chart/2(prevOutput)
  torq_setpoint/1 -> Chart/1(setpoint)
  Chart/1(output) -> output/1  "output"

== system LDM_Controller/Parallel-Hybird Controller/Decel PI controler/PI controller/Anti-windup ==
  I : Inport
  postOutput : Inport  Port=2
  preOutput : Inport  Port=3
  Gain : Gain  Gain=3  SaturateOnIntegerOverflow=on  OutDataTypeStr=Inherit: Same as input  ParamDataTypeStr=Inherit: Same as input
  Minus : Sum  Inputs=|+-
  Minus1 : Sum  Inputs=|++
  I_out : Outport
  wires:
  I/1 -> Minus1/2
  preOutput/1 -> Minus/2
  Minus1/1 -> I_out/1
  Gain/1 -> Minus1/1
  postOutput/1 -> Minus/1
  Minus/1 -> Gain/1

== system LDM_Controller/Switch-Hybird Controller/Decel PI controler/PI controller/Anti-windup ==
  I : Inport
  postOutput : Inport  Port=2
  preOutput : Inport  Port=3
  Gain : Gain  Gain=2  SaturateOnIntegerOverflow=on  OutDataTypeStr=Inherit: Same as input  ParamDataTypeStr=Inherit: Same as input
  Minus : Sum  Inputs=|+-
  Minus1 : Sum  Inputs=|++
  I_out : Outport
  wires:
  Minus/1 -> Gain/1
  postOutput/1 -> Minus/1
  Gain/1 -> Minus1/1
  Minus1/1 -> I_out/1
  preOutput/1 -> Minus/2
  I/1 -> Minus1/2

== stateflow chart LDM_Controller/Switch-Hybird Controller/VehOritArb ==
  state Normal
    state Park
      V_LDM_stVehFwBw_en = LDMVehFwBw_en_t.Park;
    state Backward
      V_LDM_stVehFwBw_en = LDMVehFwBw_en_t.Backward;
    state Null
      V_LDM_stVehFwBw_en = LDMVehFwBw_en_t.Null;
    state Forward
      V_LDM_stVehFwBw_en = LDMVehFwBw_en_t.Forward;
    (default) -> (junction 33)
    (junction 33) -> Park [order 1] : [V_DBR_stTrShftLvrPos_en == TrShftLvrPos_en_t.ParkRange]
    Park -> Normal : [V_DBR_stTrShftLvrPos_en ~= TrShftLvrPos_en_t.ParkRange]
    (junction 33) -> (junction 44) [order 2]
    (junction 44) -> Backward [order 1] : [V_DBR_stTrShftLvrPos_en == TrShftLvrPos_en_t.ReverseRange]
    Backward -> Normal : [V_DBR_stTrShftLvrPos_en ~= TrShftLvrPos_en_t.ReverseRange]
    (junction 44) -> (junction 48) [order 2]
    (junction 48) -> Null [order 1] : [V_DBR_stTrShftLvrPos_en == TrShftLvrPos_en_t.BetweenRange || ...
        | V_DBR_stTrShftLvrPos_en == TrShftLvrPos_en_t.NeutralRange || ...
        | V_DBR_stTrShftLvrPos_en == TrShftLvrPos_en_t.Unknown]
    Null -> Normal : [V_DBR_stTrShftLvrPos_en ~= TrShftLvrPos_en_t.BetweenRange && ...
        | V_DBR_stTrShftLvrPos_en ~= TrShftLvrPos_en_t.NeutralRange && ...
        | V_DBR_stTrShftLvrPos_en ~= TrShftLvrPos_en_t.Unknown]
    (junction 48) -> (junction 41) [order 2]
    Forward -> Normal : [V_DBR_stTrShftLvrPos_en <4 || V_DBR_stTrShftLvrPos_en >11]
    (junction 41) -> Forward : % V_DBR_stTrShftLvrPos_en >=4 && V_DBR_stTrShftLvrPos_en<=11
  state Error
    V_LDM_stVehFwBw_en = LDMVehFwBw_en_t.Error;
  (default) -> (junction 35)
  (junction 35) -> Normal [order 1] : [V_DBR_vldTrShftLvrPosVD_bl == false]
  (junction 35) -> Error [order 2] : % V_DBR_vldTrShftLvrPosVD_bl == true
  Error -> Normal : [V_DBR_vldTrShftLvrPosVD_bl == false]
  Normal -> Error : [V_DBR_vldTrShftLvrPosVD_bl == true]
  data: V_DBR_vldTrShftLvrPosVD_bl input boolean; V_DBR_stTrShftLvrPos_en input Enum: TrShftLvrPos_en_t; V_LDM_stVehFwBw_en output Enum: LDMVehFwBw_en_t

== stateflow chart LDM_Controller/Switch-Hybird Controller/Decel open-loop controler/Subsystem/Chart ==
  state Initial
    output = prevOutput;
  state openLoopSetpointFollow
    if prevOutput > setpoint + 2*K_LDM_torqOLCtrlerDecRate
    output = output - K_LDM_torqOLCtrlerDecRate;
    elseif prevOutput < setpoint - 2*K_LDM_torqOLCtrlerIncRate
    output = output +K_LDM_torqOLCtrlerIncRate;
    else
    output = prevOutput;
    end
  (default) -> Initial
  Initial -> openLoopSetpointFollow
  data: setpoint input; K_LDM_torqOLCtrlerIncRate parameter; K_LDM_torqOLCtrlerDecRate parameter; prevOutput input; output output
